simulink model "Dashboard"  (R2023b)
settings: Solver=VariableStepAuto  StartTime=0.0  StopTime=10.0  RelTol=1e-3
model workspace (MAT data in the model file):
  aa = 1
settings Model: Creator=MURTI  LastModifiedBy=MURTI

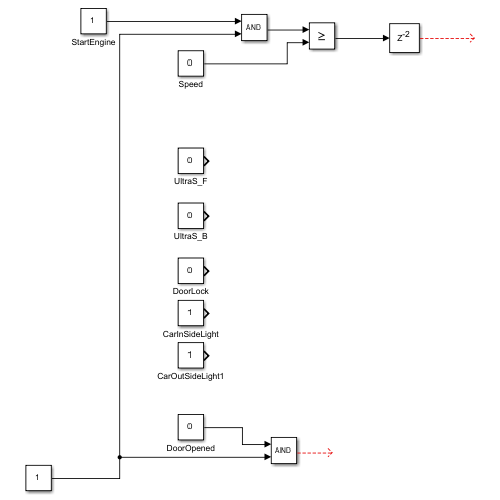
[thumbnail: Simulink's stored preview of the top-level diagram]
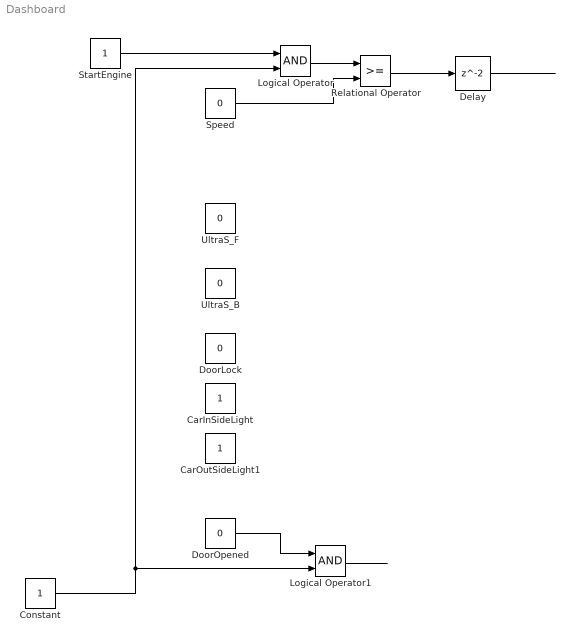
== system Dashboard ==
  CarInSideLight : Constant
  CarOutSideLight1 : Constant
  Constant : Constant
  Delay : Delay
  DoorLock : Constant  Value=0
  DoorOpened : Constant  Value=0
  Logical Operator : Logic  AllPortsSameDT=off  OutDataTypeStr=boolean
  Logical Operator1 : Logic  AllPortsSameDT=off  OutDataTypeStr=boolean
  Relational Operator : RelationalOperator  OutDataTypeStr=boolean  RndMeth=Simplest  InputSameDT=off
  Speed : Constant  Value=0
  StartEngine : Constant
  UltraS_B : Constant  Value=0
  UltraS_F : Constant  Value=0
  wires:
  StartEngine/1 -> Logical Operator/1
  Constant/1 -> Logical Operator/2, Logical Operator1/2
  Logical Operator/1 -> Relational Operator/1
  DoorOpened/1 -> Logical Operator1/1
  Logical Operator1/1 -> ?
  Speed/1 -> Relational Operator/2
  Relational Operator/1 -> Delay/1
  Delay/1 -> ?
